simulink model "coluna_sim"  (R2025a)
settings: Solver=VariableStepAuto  StartTime=0.0  StopTime=10000  MaxStep=1  RelTol=1e-3
values from neighbouring files (symbols this model uses):
  p = block.DialogPrm(1).Data    [coluna_sfun.m]
libraries: slpidlib x2
settings Model: Creator=hdafg  LastModifiedBy=hdafg
settings DataIOCC: ExternalInput=inputSignal  OutputSaveName=simData
settings DebuggingCC: BusObjectLabelMismatch=none

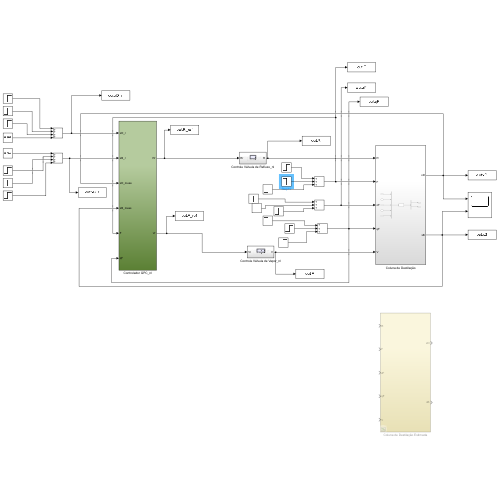
[thumbnail: Simulink's stored preview of the top-level diagram]
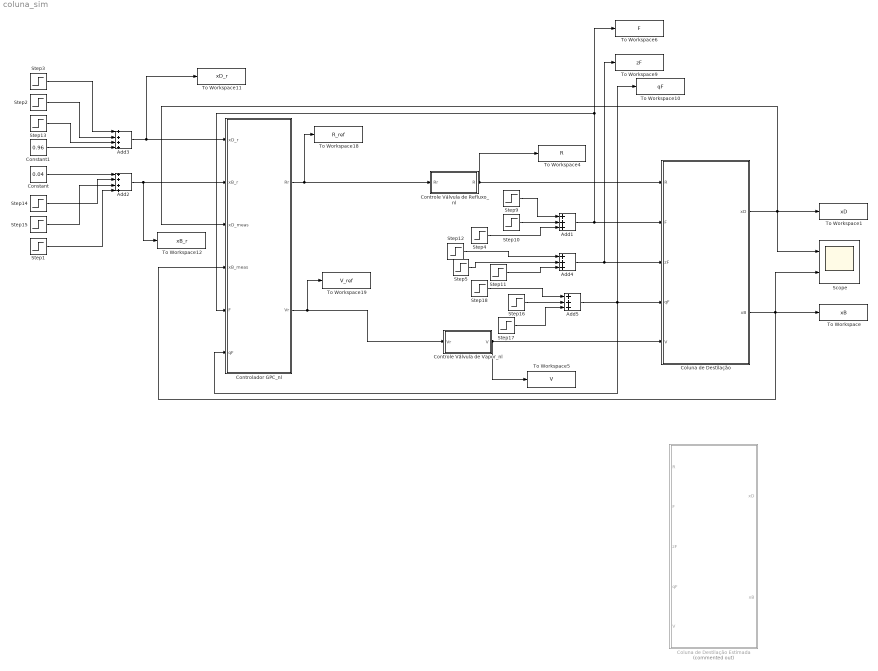
== system coluna_sim ==
  Add1 : Sum  Inputs=+++
  Add2 : Sum  Inputs=++++
  Add3 : Sum  Inputs=++++
  Add4 : Sum  Inputs=+++
  Add5 : Sum  Inputs=+++
  Coluna de Destilação : Subsystem
  Coluna de Destilação Estimada : Subsystem  Commented=on
  Constant : Constant  Value=0.04
  Constant1 : Constant  Value=0.96
  Controlador GPC_nl : Subsystem
  Controle Válvula de Refluxo_nl : Subsystem
  Controle Válvula de Vapor_nl : Subsystem
  Scope : Scope  NumInputPorts=2
      settings: ActiveDisplayYMinimum=-0.11799999999999997  ActiveDisplayYMaximum=1.1219999999999999
  Step1 : Step  Time=3500  After=0  SampleTime=0
  Step10 : Step  Time=5800  After=-0.1  SampleTime=0
  Step11 : Step  Time=3500  After=0  SampleTime=0
  Step12 : Step  Time=2800  Before=0.5  After=0.55  SampleTime=0
  Step13 : Step  Time=2000  After=0  SampleTime=0
  Step14 : Step  Time=2500  After=0  SampleTime=0
  Step15 : Step  Time=3000  After=0  SampleTime=0
  Step16 : Step  Time=1800  After=0.1  SampleTime=0
  Step17 : Step  Time=5000  After=0  SampleTime=0
  Step18 : Step  Time=800  Before=1  After=0.9  SampleTime=0
  Step2 : Step  Time=1500  After=0  SampleTime=0
  Step3 : Step  Time=2000  After=0  SampleTime=0
  Step4 : Step  Time=2000  After=0  SampleTime=0
  Step5 : Step  Time=3800  After=-0.05  SampleTime=0
  Step9 : Step  Time=4800  Before=1  After=1.1  SampleTime=0
  To Workspace : ToWorkspace  VariableName=xB  SaveFormat=Timeseries  SampleTime=-1
  To Workspace1 : ToWorkspace  VariableName=xD  SaveFormat=Timeseries  SampleTime=-1
  To Workspace10 : ToWorkspace  VariableName=qF  SaveFormat=Timeseries  SampleTime=-1
  To Workspace11 : ToWorkspace  VariableName=xD_r  SaveFormat=Timeseries  SampleTime=-1
  To Workspace12 : ToWorkspace  VariableName=xB_r  SaveFormat=Timeseries  SampleTime=-1
  To Workspace18 : ToWorkspace  VariableName=R_ref  SaveFormat=Timeseries  SampleTime=-1
  To Workspace19 : ToWorkspace  VariableName=V_ref  SaveFormat=Timeseries  SampleTime=-1
  To Workspace4 : ToWorkspace  VariableName=R  SaveFormat=Timeseries  SampleTime=-1
  To Workspace5 : ToWorkspace  VariableName=V  SaveFormat=Timeseries  SampleTime=-1
  To Workspace6 : ToWorkspace  VariableName=F  SaveFormat=Timeseries  SampleTime=-1
  To Workspace9 : ToWorkspace  VariableName=zF  SaveFormat=Timeseries  SampleTime=-1
  wires:
  Controle Válvula de Vapor_nl/1(V) -> Coluna de Destilação/5(V), To Workspace5/1
  Controle Válvula de Refluxo_nl/1(R) -> Coluna de Destilação/1(R), To Workspace4/1
  Add1/1 -> Coluna de Destilação/2(F), Controlador GPC_nl/5(F), To Workspace6/1
  Add4/1 -> Coluna de Destilação/3(zF), To Workspace9/1
  Add5/1 -> Coluna de Destilação/4(qF), Controlador GPC_nl/6(qF), To Workspace10/1
  Add2/1 -> To Workspace12/1, Controlador GPC_nl/2(xB_r)
  Add3/1 -> To Workspace11/1, Controlador GPC_nl/1(xD_r)
  Coluna de Destilação/1(xD) -> Scope/1, Controlador GPC_nl/3(xD_meas), To Workspace1/1
  Coluna de Destilação/2(xB) -> Scope/2, Controlador GPC_nl/4(xB_meas), To Workspace/1
  Controlador GPC_nl/1(Rr) -> Controle Válvula de Refluxo_nl/1(Rr), To Workspace18/1
  Controlador GPC_nl/2(Vr) -> To Workspace19/1, Controle Válvula de Vapor_nl/1(Vr)
  Step2/1 -> Add3/2
  Step13/1 -> Add3/3
  Step3/1 -> Add3/1
  Step10/1 -> Add1/2
  Step4/1 -> Add1/3
  Step9/1 -> Add1/1
  Step12/1 -> Add4/1
  Step11/1 -> Add4/3
  Step5/1 -> Add4/2
  Step18/1 -> Add5/1
  Step17/1 -> Add5/3
  Step16/1 -> Add5/2
  Step14/1 -> Add2/2
  Step15/1 -> Add2/3
  Step1/1 -> Add2/4
  Constant/1 -> Add2/1
  Constant1/1 -> Add3/4

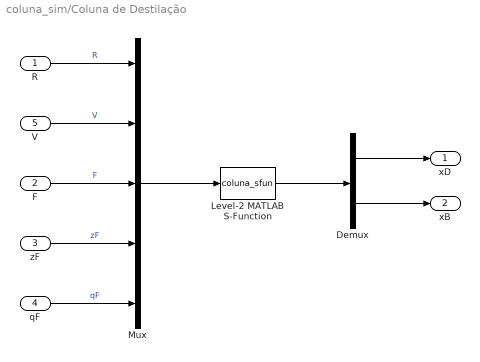
== system coluna_sim/Coluna de Destilação ==
  R : Inport
  F : Inport  Port=2
  zF : Inport  Port=3
  qF : Inport  Port=4
  V : Inport  Port=5
  Demux : Demux  Outputs=2
  Level-2 MATLAB S-Function : M-S-Function  FunctionName=coluna_sfun  Parameters=p
  Mux : Mux  Inputs=5
  xD : Outport
  xB : Outport  Port=2
  wires:
  F/1 -> Mux/3  "F"
  qF/1 -> Mux/5  "qF"
  R/1 -> Mux/1  "R"
  zF/1 -> Mux/4  "zF"
  Mux/1 -> Level-2 MATLAB S-Function/1
  Level-2 MATLAB S-Function/1 -> Demux/1
  V/1 -> Mux/2  "V"
  Demux/2 -> xB/1
  Demux/1 -> xD/1

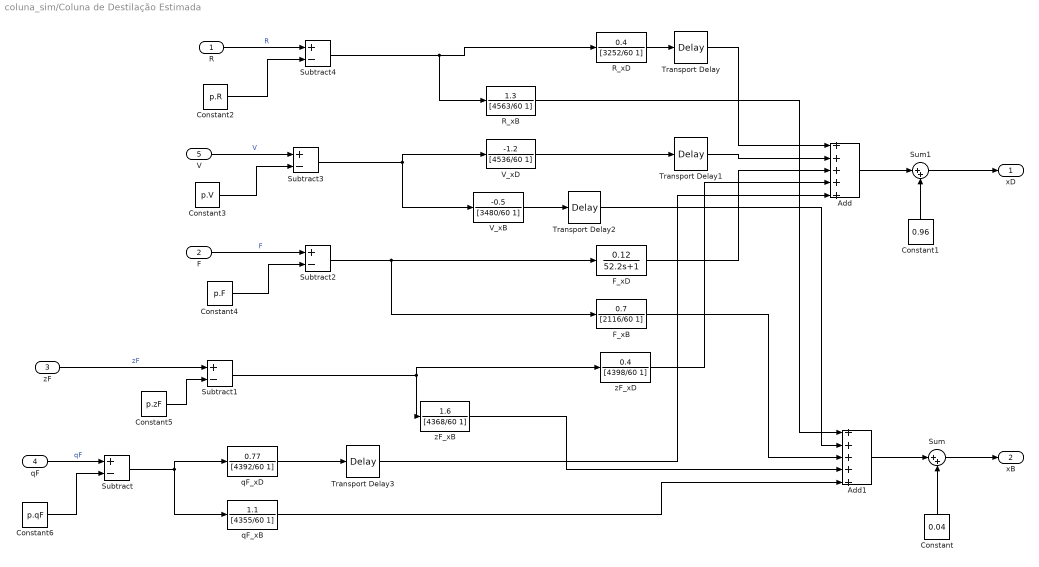
== system coluna_sim/Coluna de Destilação Estimada ==
  R : Inport
  F : Inport  Port=2
  zF : Inport  Port=3
  qF : Inport  Port=4
  V : Inport  Port=5
  Add : Sum  Inputs=+++++
  Add1 : Sum  Inputs=+++++
  Constant : Constant  Value=0.04
  Constant1 : Constant  Value=0.96
  Constant2 : Constant  Value=p.R
  Constant3 : Constant  Value=p.V
  Constant4 : Constant  Value=p.F
  Constant5 : Constant  Value=p.zF
  Constant6 : Constant  Value=p.qF
  F_xB : TransferFcn  Numerator=0.7  Denominator=[2116/60 1]
  F_xD : TransferFcn  Numerator=0.12  Denominator=[52.2 1]
  R_xB : TransferFcn  Numerator=1.3  Denominator=[4563/60 1]
  R_xD : TransferFcn  Numerator=[0.4]  Denominator=[3252/60 1]
  Subtract{,1..4} (5 alike) : Sum  Inputs=+-
  Sum : Sum  Inputs=|++
  Sum1 : Sum  Inputs=|++
  Transport Delay : TransportDelay  DelayTime=9.36/60
  Transport Delay1 : TransportDelay  DelayTime=9.6/60
  Transport Delay2 : TransportDelay  DelayTime=9.6
  Transport Delay3 : TransportDelay  DelayTime=17.1/60
  V_xB : TransferFcn  Numerator=-0.5  Denominator=[3480/60 1]
  V_xD : TransferFcn  Numerator=-1.2  Denominator=[4536/60 1]
  qF_xB : TransferFcn  Numerator=1.1  Denominator=[4355/60 1]
  qF_xD : TransferFcn  Numerator=0.77  Denominator=[4392/60 1]
  zF_xB : TransferFcn  Numerator=1.6  Denominator=[4368/60 1]
  zF_xD : TransferFcn  Numerator=0.4  Denominator=[4398/60 1]
  xD : Outport
  xB : Outport  Port=2
  wires:
  F/1 -> Subtract2/1  "F"
  zF/1 -> Subtract1/1  "zF"
  R_xD/1 -> Transport Delay/1
  V_xD/1 -> Transport Delay1/1
  F_xD/1 -> Add/3
  zF_xD/1 -> Add/4
  qF_xD/1 -> Transport Delay3/1
  R_xB/1 -> Add1/1
  V_xB/1 -> Transport Delay2/1
  F_xB/1 -> Add1/3
  zF_xB/1 -> Add1/4
  qF_xB/1 -> Add1/5
  Add1/1 -> Sum/1
  Sum/1 -> xB/1
  Constant/1 -> Sum/2
  Add/1 -> Sum1/1
  Sum1/1 -> xD/1
  Constant1/1 -> Sum1/2
  Transport Delay/1 -> Add/1
  Transport Delay1/1 -> Add/2
  Transport Delay2/1 -> Add1/2
  Transport Delay3/1 -> Add/5
  qF/1 -> Subtract/1  "qF"
  Subtract/1 -> qF_xB/1, qF_xD/1
  Subtract1/1 -> zF_xB/1, zF_xD/1
  Subtract2/1 -> F_xB/1, F_xD/1
  V/1 -> Subtract3/1  "V"
  Subtract3/1 -> V_xB/1, V_xD/1
  R/1 -> Subtract4/1  "R"
  Subtract4/1 -> R_xB/1, R_xD/1
  Constant2/1 -> Subtract4/2
  Constant3/1 -> Subtract3/2
  Constant4/1 -> Subtract2/2
  Constant5/1 -> Subtract1/2
  Constant6/1 -> Subtract/2

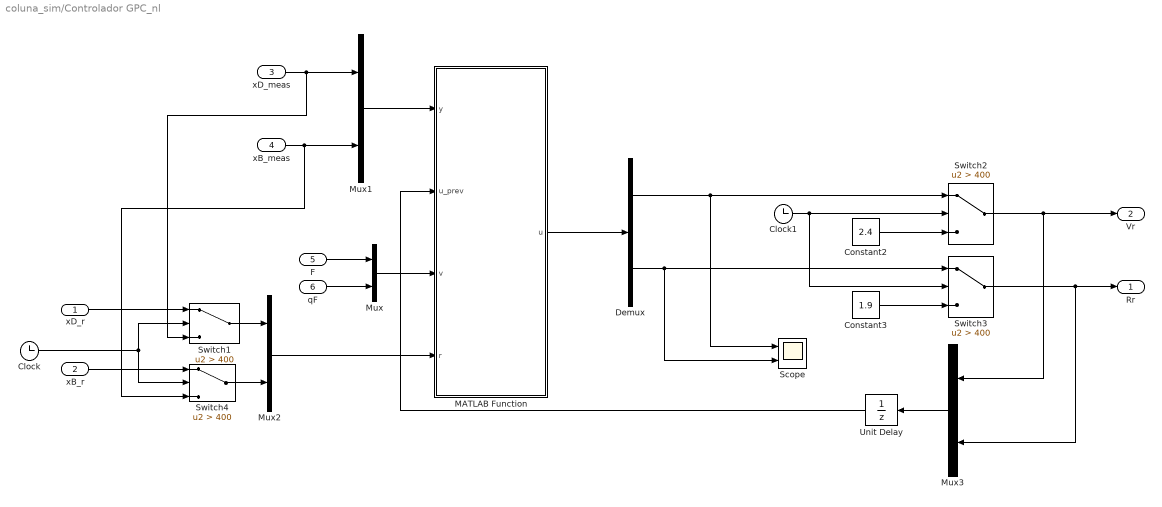
== system coluna_sim/Controlador GPC_nl ==
  xD_r : Inport
  xB_r : Inport  Port=2
  xD_meas : Inport  Port=3
  xB_meas : Inport  Port=4
  F : Inport  Port=5
  qF : Inport  Port=6
  Clock : Clock
  Clock1 : Clock
  Constant2 : Constant  Value=2.4
  Constant3 : Constant  Value=1.9
  Demux : Demux  Outputs=2
  MATLAB Function : MATLAB Function  TreatAsAtomicUnit=on
  Mux{,1..3} (4 alike) : Mux  Inputs=2
  Scope : Scope  NumInputPorts=2
      settings: ActiveDisplayYMinimum=-0.30135374803202258  ActiveDisplayYMaximum=2.7121837322882039  DataLoggingVariableName=ScopeData2
  Switch{1..4} (4 alike) : Switch  Criteria=u2 > Threshold  Threshold=400  SaturateOnIntegerOverflow=off  InputSameDT=off
  Unit Delay : UnitDelay  HasFrameUpgradeWarning=on
  Rr : Outport
  Vr : Outport  Port=2
  wires:
  Mux/1 -> MATLAB Function/3(v)
  F/1 -> Mux/1
  qF/1 -> Mux/2
  Mux2/1 -> MATLAB Function/4(r)
  Mux1/1 -> MATLAB Function/1(y)
  MATLAB Function/1(u) -> Demux/1
  Unit Delay/1 -> MATLAB Function/2(u_prev)
  Switch2/1 -> Mux3/1, Vr/1
  Constant2/1 -> Switch2/3
  Clock1/1 -> Switch3/2, Switch2/2
  Constant3/1 -> Switch3/3
  Switch3/1 -> Mux3/2, Rr/1
  Demux/2 -> Scope/2, Switch3/1
  Demux/1 -> Scope/1, Switch2/1
  Mux3/1 -> Unit Delay/1
  xB_meas/1 -> Switch4/3, Mux1/2
  xD_meas/1 -> Switch1/3, Mux1/1
  Clock/1 -> Switch1/2, Switch4/2
  Switch1/1 -> Mux2/1
  Switch4/1 -> Mux2/2
  xD_r/1 -> Switch1/1
  xB_r/1 -> Switch4/1

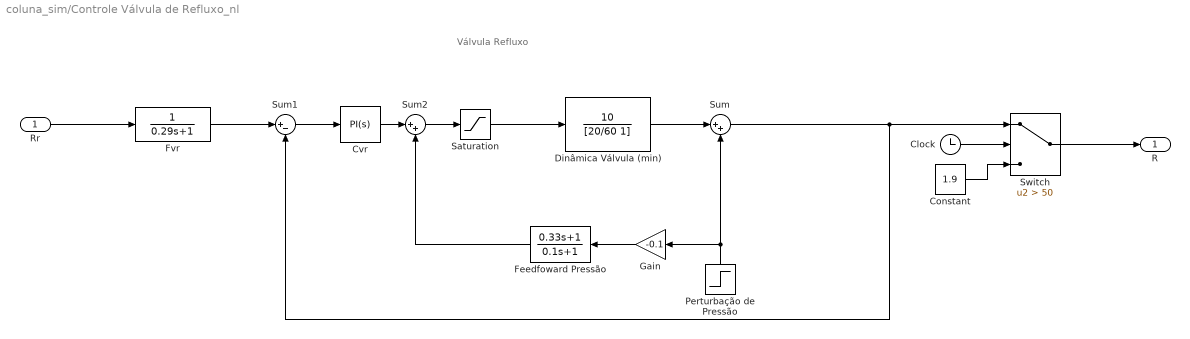
== system coluna_sim/Controle Válvula de Refluxo_nl ==
  note: Válvula Refluxo
  Rr : Inport
  Clock : Clock
  Constant : Constant  Value=1.9
  Cvr : slpidlib/PID Controller  Controller=PI  Form=Parallel  TimeDomain=Continuous-time  UseExternalTs=off  SampleTime=-1  IntegratorMethod=Forward Euler  FilterMethod=Forward Euler  ControllerParametersSource=internal  P=0.22  I=0.768  UseKiTs=off  D=0  UseExternalDerivativeSource=off  N=100  UseFilter=on  TunerSelectOption=Transfer Function Based (PID Tuner App)  InitialConditionSource=internal  InitialConditionForIntegrator=0  InitialConditionForFilter=0  DifferentiatorICPrevScaledInput=0  ExternalReset=none  TrackingMode=off  Kt=1  LimitOutput=on  SatLimitsSource=internal  UpperSaturationLimit=1  LowerSaturationLimit=0  LinearizeAsGain=on  AntiWindupMode=back-calculation  Kb=1/0.29  LimitIntegrator=off  UpperIntegratorSaturationLimit=inf  LowerIntegratorSaturationLimit=-inf  POutMin=[]  POutMax=[]  IOutMin=[]  IOutMax=[]  DOutMin=[]  DOutMax=[]  NOutMin=[]  NOutMax=[]  SumOutMin=[]  SumOutMax=[]  SaturationOutMin=[]  SaturationOutMax=[]  PParamMin=[]  PParamMax=[]  IParamMin=[]  IParamMax=[]  DParamMin=[]  DParamMax=[]  NParamMin=[]  NParamMax=[]  KbParamMin=[]  KbParamMax=[]  KtParamMin=[]  KtParamMax=[]  KbOutMin=[]  KbOutMax=[]  KtOutMin=[]  KtOutMax=[]  IntegratorOutMin=[]  IntegratorOutMax=[]  FilterOutMin=[]  FilterOutMax=[]  SumI1OutMin=[]  SumI1OutMax=[]  SumI2OutMin=[]  SumI2OutMax=[]  SumI3OutMin=[]  SumI3OutMax=[]  SumI4OutMin=[]  SumI4OutMax=[]  SumDOutMin=[]  SumDOutMax=[]  DifferentiatorOutMin=[]  DifferentiatorOutMax=[]  FilterDiffOutCoefMin=[]  FilterDiffOutCoefMax=[]  ReciprocalOutMin=[]  ReciprocalOutMax=[]  SumDenOutMin=[]  SumDenOutMax=[]  SumNumOutMin=[]  SumNumOutMax=[]  DivideOutMin=[]  DivideOutMax=[]  UdiffTsProdOutMin=[]  UdiffTsProdOutMax=[]  NTsProdOutMin=[]  NTsProdOutMax=[]  UintegralTsProdOutMin=[]  UintegralTsProdOutMax=[]  UngainTsProdOutMin=[]  UngainTsProdOutMax=[]  ClampingZeroOutDataTypeStr=Inherit: Inherit via back propagation  ClampingZeroOutMin=[]  ClampingZeroOutMax=[]  FilterDenConstantOutDataTypeStr=Inherit: Inherit via back propagation  FilterDenConstantOutMin=[]  FilterDenConstantOutMax=[]  PCopyOutDataTypeStr=Inherit: Inherit via back propagation  PCopyOutMin=[]  PCopyOutMax=[]  NCopyOutDataTypeStr=Inherit: Inherit via back propagation  NCopyOutMin=[]  NCopyOutMax=[]  IntegratorContinuousStateAttributes=''  IntegratorStateMustResolveToSignalObject=off  IntegratorRTWStateStorageClass=Auto  FilterContinuousStateAttributes=''  FilterStateMustResolveToSignalObject=off  FilterRTWStateStorageClass=Auto  ParallelPVariant=InternalParameters  IdealPVariant=Disabled  IVariant=InternalParameters  DVariant=Disabled  IntegratorVariant=Continuous  SatVariant=Enabled  AWVariant=BackCalculation  PCopyVariant=Disabled  TRVariant=Disabled  FdbkBlocksVariant=Forward  IdealPFdbkVariant=Disabled  SatFdbkVariant=Disabled  DerivativeFilterVariant=Disabled  NVariant=Disabled  NCopyVariant=Disabled_SignalSpec  FilterICVariant=Disabled  IntegratorICVariant=InternalICs  ExternalResetVariant=Disabled  TRSumVariant=Passthrough  SumFdbkVariant=Disabled  SumVariant=Sum_PI  TsampFilterVariant=InternalTs  TsampNgainVariant=Passthrough  TsampIntegralVariant=Disabled_SignalSpec  ExternalSaturationOutDataTypeStr=Inherit: Same as second input  DerivativeSourceVariant=Disabled  PreIntVariant=InternalPreInt
  Dinâmica Válvula (min) : TransferFcn  Numerator=[10]  Denominator=[20/60 1]
  Feedfoward Pressão : TransferFcn  Numerator=[0.33 1]  Denominator=[0.1 1]
  Fvr : TransferFcn  Denominator=[0.29 1]
  Gain : Gain  Gain=-0.1
  Perturbação de Pressão : Step  Time=10  After=-1  SampleTime=0
  Saturation : Saturate  UpperLimit=1  LowerLimit=0
  Sum : Sum  Inputs=|++
  Sum1 : Sum  Inputs=|+-
  Sum2 : Sum  Inputs=|++
  Switch : Switch  Criteria=u2 > Threshold  Threshold=50  SaturateOnIntegerOverflow=off  InputSameDT=off
  R : Outport
  wires:
  Cvr/1 -> Sum2/1
  Saturation/1 -> Dinâmica Válvula (min)/1
  Feedfoward Pressão/1 -> Sum2/2
  Perturbação de Pressão/1 -> Gain/1, Sum/2
  Sum1/1 -> Cvr/1
  Gain/1 -> Feedfoward Pressão/1
  Dinâmica Válvula (min)/1 -> Sum/1
  Sum2/1 -> Saturation/1
  Fvr/1 -> Sum1/1
  Sum/1 -> Sum1/2, Switch/1
  Rr/1 -> Fvr/1
  Clock/1 -> Switch/2
  Switch/1 -> R/1
  Constant/1 -> Switch/3

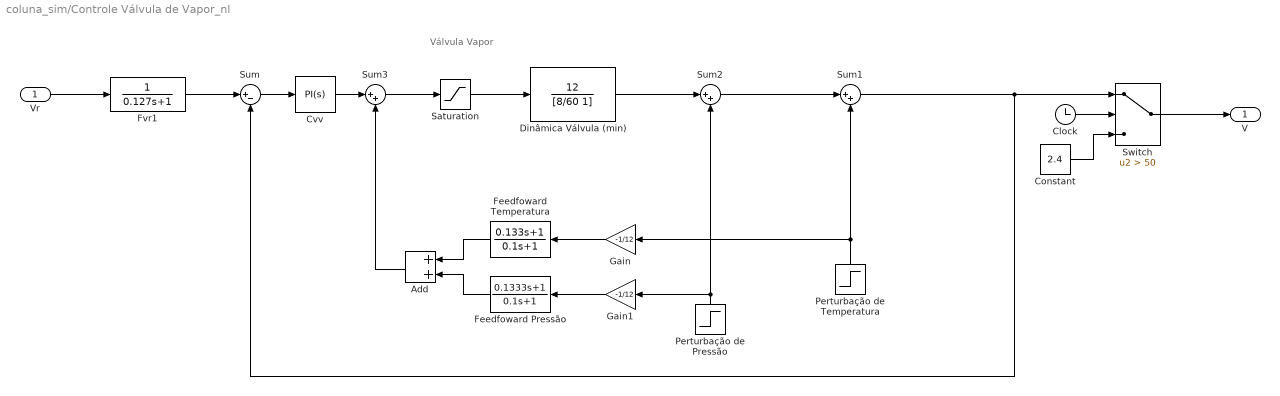
== system coluna_sim/Controle Válvula de Vapor_nl ==
  note: Válvula Vapor
  Vr : Inport
  Add : Sum
  Clock : Clock
  Constant : Constant  Value=2.4
  Cvv : slpidlib/PID Controller  Controller=PI  Form=Parallel  TimeDomain=Continuous-time  UseExternalTs=off  SampleTime=-1  IntegratorMethod=Forward Euler  FilterMethod=Forward Euler  ControllerParametersSource=internal  P=0.34  I=2.677  UseKiTs=off  D=0  UseExternalDerivativeSource=off  N=100  UseFilter=on  TunerSelectOption=Transfer Function Based (PID Tuner App)  InitialConditionSource=internal  InitialConditionForIntegrator=0  InitialConditionForFilter=0  DifferentiatorICPrevScaledInput=0  ExternalReset=none  TrackingMode=off  Kt=1  LimitOutput=on  SatLimitsSource=internal  UpperSaturationLimit=1  LowerSaturationLimit=0  LinearizeAsGain=on  AntiWindupMode=back-calculation  Kb=1/0.127  LimitIntegrator=off  UpperIntegratorSaturationLimit=inf  LowerIntegratorSaturationLimit=-inf  POutMin=[]  POutMax=[]  IOutMin=[]  IOutMax=[]  DOutMin=[]  DOutMax=[]  NOutMin=[]  NOutMax=[]  SumOutMin=[]  SumOutMax=[]  SaturationOutMin=[]  SaturationOutMax=[]  PParamMin=[]  PParamMax=[]  IParamMin=[]  IParamMax=[]  DParamMin=[]  DParamMax=[]  NParamMin=[]  NParamMax=[]  KbParamMin=[]  KbParamMax=[]  KtParamMin=[]  KtParamMax=[]  KbOutMin=[]  KbOutMax=[]  KtOutMin=[]  KtOutMax=[]  IntegratorOutMin=[]  IntegratorOutMax=[]  FilterOutMin=[]  FilterOutMax=[]  SumI1OutMin=[]  SumI1OutMax=[]  SumI2OutMin=[]  SumI2OutMax=[]  SumI3OutMin=[]  SumI3OutMax=[]  SumI4OutMin=[]  SumI4OutMax=[]  SumDOutMin=[]  SumDOutMax=[]  DifferentiatorOutMin=[]  DifferentiatorOutMax=[]  FilterDiffOutCoefMin=[]  FilterDiffOutCoefMax=[]  ReciprocalOutMin=[]  ReciprocalOutMax=[]  SumDenOutMin=[]  SumDenOutMax=[]  SumNumOutMin=[]  SumNumOutMax=[]  DivideOutMin=[]  DivideOutMax=[]  UdiffTsProdOutMin=[]  UdiffTsProdOutMax=[]  NTsProdOutMin=[]  NTsProdOutMax=[]  UintegralTsProdOutMin=[]  UintegralTsProdOutMax=[]  UngainTsProdOutMin=[]  UngainTsProdOutMax=[]  ClampingZeroOutDataTypeStr=Inherit: Inherit via back propagation  ClampingZeroOutMin=[]  ClampingZeroOutMax=[]  FilterDenConstantOutDataTypeStr=Inherit: Inherit via back propagation  FilterDenConstantOutMin=[]  FilterDenConstantOutMax=[]  PCopyOutDataTypeStr=Inherit: Inherit via back propagation  PCopyOutMin=[]  PCopyOutMax=[]  NCopyOutDataTypeStr=Inherit: Inherit via back propagation  NCopyOutMin=[]  NCopyOutMax=[]  IntegratorContinuousStateAttributes=''  IntegratorStateMustResolveToSignalObject=off  IntegratorRTWStateStorageClass=Auto  FilterContinuousStateAttributes=''  FilterStateMustResolveToSignalObject=off  FilterRTWStateStorageClass=Auto  ParallelPVariant=InternalParameters  IdealPVariant=Disabled  IVariant=InternalParameters  DVariant=Disabled  IntegratorVariant=Continuous  SatVariant=Enabled  AWVariant=BackCalculation  PCopyVariant=Disabled  TRVariant=Disabled  FdbkBlocksVariant=Forward  IdealPFdbkVariant=Disabled  SatFdbkVariant=Disabled  DerivativeFilterVariant=Disabled  NVariant=Disabled  NCopyVariant=Disabled_SignalSpec  FilterICVariant=Disabled  IntegratorICVariant=InternalICs  ExternalResetVariant=Disabled  TRSumVariant=Passthrough  SumFdbkVariant=Disabled  SumVariant=Sum_PI  TsampFilterVariant=InternalTs  TsampNgainVariant=Passthrough  TsampIntegralVariant=Disabled_SignalSpec  ExternalSaturationOutDataTypeStr=Inherit: Same as second input  DerivativeSourceVariant=Disabled  PreIntVariant=InternalPreInt
  Dinâmica Válvula (min) : TransferFcn  Numerator=[12]  Denominator=[8/60 1]
  Feedfoward Pressão : TransferFcn  Numerator=[0.1333 1]  Denominator=[0.1 1]
  Feedfoward Temperatura : TransferFcn  Numerator=[0.133 1]  Denominator=[0.1 1]
  Fvr1 : TransferFcn  Denominator=[0.127 1]
  Gain : Gain  Gain=-1/12
  Gain1 : Gain  Gain=-1/12
  Perturbação de Pressão : Step  Time=9  After=0.5  SampleTime=0
  Perturbação de Temperatura : Step  Time=12  After=0.8  SampleTime=0
  Saturation : Saturate  UpperLimit=1  LowerLimit=0
  Sum : Sum  Inputs=|+-
  Sum1 : Sum  Inputs=|++
  Sum2 : Sum  Inputs=|++
  Sum3 : Sum  Inputs=|++
  Switch : Switch  Criteria=u2 > Threshold  Threshold=50  SaturateOnIntegerOverflow=off  InputSameDT=off
  V : Outport
  wires:
  Dinâmica Válvula (min)/1 -> Sum2/1
  Feedfoward Pressão/1 -> Add/2
  Perturbação de Pressão/1 -> Sum2/2, Gain1/1
  Sum/1 -> Cvv/1
  Cvv/1 -> Sum3/1
  Add/1 -> Sum3/2
  Feedfoward Temperatura/1 -> Add/1
  Sum1/1 -> Sum/2, Switch/1
  Vr/1 -> Fvr1/1
  Gain1/1 -> Feedfoward Pressão/1
  Saturation/1 -> Dinâmica Válvula (min)/1
  Gain/1 -> Feedfoward Temperatura/1
  Perturbação de Temperatura/1 -> Gain/1, Sum1/2
  Sum3/1 -> Saturation/1
  Sum2/1 -> Sum1/1
  Fvr1/1 -> Sum/1
  Switch/1 -> V/1
  Clock/1 -> Switch/2
  Constant/1 -> Switch/3

== matlab function coluna_sim/Controlador GPC_nl/MATLAB Function ==
  settings: updateMethod=DISCRETE  sampleTime=1
  data: y input; u output; u_prev input; v input; r input
function u = GPC_Controller_Block(y, u_prev, v, r)
% Bloco de função do GPC para Simulink
% 
% Entradas:
%   y      - Saídas medidas [2x1]
%   u_prev - Entradas anteriores [2x1]
%   v      - Perturbações medidas [2x1]
%   r      - Referências [2x1]
%
% Saída:
%   u      - Entradas calculadas [2x1]

%#codegen

% Carregar dados do controlador (usar persistent para eficiência)
persistent controller_data

if isempty(controller_data)
    % Carregar na primeira execução
    data = load('GPC_MIMO_Controller_Data.mat');
    controller_data = data.controller_data;
end

% Chamar função do controlador
[u, ~, ~] = GPC_MIMO_Controller(y, u_prev, v, r, controller_data);

end
